simulink model "c_syst"  (R2015a)
settings: Solver=ode45  StartTime=0.0  StopTime=20  RelTol=1e-3
values from neighbouring files (symbols this model uses):
  A = A    [design.m]    (also in init.mat = [2.98564337206 1 0 0 0 -3.00327796547 0 1 0 0 0.709627661926)
  B = B    [design.m]    (also in init.mat = [1 0 0 0 0])
  C = [-0.0746143795197 0.142131862116 0 0 0]    [init.mat]
  D = zeros(1+length(A(:,1)),1)    [design.m]    (also in init.mat = 0)
  H = [C;eye(size(A))]    [design.m]
  Ke = -3.8587    [init.mat]
  Kp = 35.7244    [init.mat]
undefined symbols (not defined in the file or in its folder): K, M, National_Instruments, PCI
libraries: sldrtlib x2
settings Model: Creator=João  LastModifiedBy=João

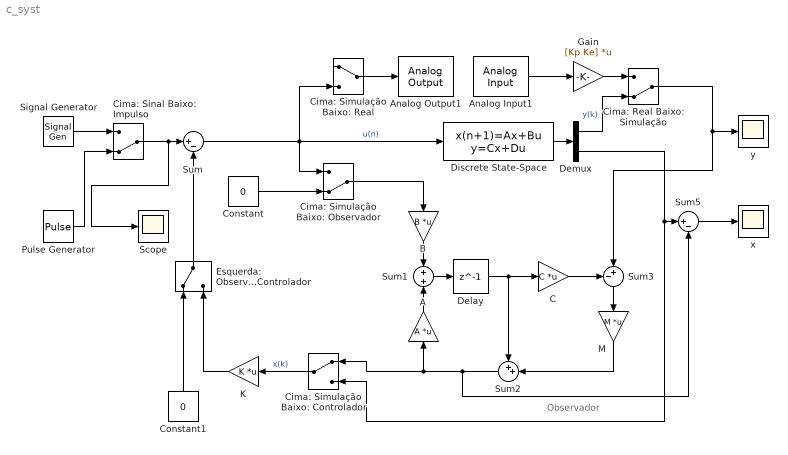
== system c_syst ==
  note: Observador
  A : Gain  Gain=A  Multiplication=Matrix(K*u) (u vector)
  Analog Input1 : sldrtlib/Analog Input  SampleTime=0.02  MaxMissedTicks=10  ShowMissedTicks=off  YieldWhenWaiting=off  DrvName=National_Instruments/PCI-6221  DrvAddress=4294967295  DrvOptions=[0 0 0 0 0]  Channels=[1 2]  RangeMode=1  VoltRange=1  DataType=1
      settings: AttributesFormatString=National Instruments\nPCI-6221 [auto]
  Analog Output1 : sldrtlib/Analog Output  SampleTime=0.02  MaxMissedTicks=10  ShowMissedTicks=off  YieldWhenWaiting=off  DrvName=National_Instruments/PCI-6221  DrvAddress=4294967295  DrvOptions=[0 0 0 0 0]  Channels=1  RangeMode=1  VoltRange=1  InitialValue=0  FinalValue=0
      settings: AttributesFormatString=National Instruments\nPCI-6221 [auto]
  B : Gain  Gain=B  Multiplication=Matrix(K*u) (u vector)
  C : Gain  Gain=C  Multiplication=Matrix(K*u) (u vector)
  Cima: Real Baixo: Simulação : ManualSwitch  CurrentSetting=0
  Cima: Simulação Baixo: Controlador : ManualSwitch
  Cima: Simulação Baixo: Observador : ManualSwitch  CurrentSetting=0
  Cima: Simulação Baixo: Real : ManualSwitch
  Cima: Sinal Baixo: Impulso : ManualSwitch  CurrentSetting=0
  Constant : Constant  Value=0
  Constant1 : Constant  Value=0
  Delay : Delay  DelayLength=1  InitialCondition=0  SampleTime=0.02
  Demux : Demux  Outputs=2
  Discrete State-Space : DiscreteStateSpace  A=A  B=B  C=H  D=D  SampleTime=0.02
  Esquerda: Observador Direita: Simulação e Controlador : ManualSwitch
  Gain : Gain  Gain=[Kp Ke]  Multiplication=Matrix(K*u) (u vector)
  K : Gain  Gain=K  Multiplication=Matrix(K*u) (u vector)
  M : Gain  Gain=M  Multiplication=Matrix(K*u) (u vector)
  Pulse Generator : DiscretePulseGenerator  PulseType=Time based  Period=20  PhaseDelay=2
  Scope : Scope
      settings: SampleInput=on
  Signal Generator : SignalGenerator  Units=rad/sec
  Sum : Sum  Inputs=|+-
  Sum1 : Sum  Inputs=+|+
  Sum2 : Sum  Inputs=++|
  Sum3 : Sum  Inputs=-+|
  Sum5 : Sum  Inputs=|+-
  x : Scope
      settings: SaveName=ScopeData2  SampleInput=on
  y : Scope
      settings: SampleInput=on
  wires:
  Sum/1 -> Cima: Simulação Baixo: Real/2, Cima: Simulação Baixo: Observador/1, Discrete State-Space/1  "u(n)"
  B/1 -> Sum1/1
  Sum1/1 -> Delay/1
  Sum2/1 -> Sum5/2, A/1, Cima: Simulação Baixo: Controlador/1
  A/1 -> Sum1/2
  Delay/1 -> C/1, Sum2/1
  C/1 -> Sum3/1
  Sum3/1 -> M/1
  M/1 -> Sum2/2
  Discrete State-Space/1 -> Demux/1
  Cima: Simulação Baixo: Controlador/1 -> K/1  "x(k)"
  Demux/2 -> Sum5/1, Cima: Simulação Baixo: Controlador/2
  Cima: Simulação Baixo: Observador/1 -> B/1
  Constant/1 -> Cima: Simulação Baixo: Observador/2
  Esquerda: Observador Direita: Simulação e Controlador/1 -> Sum/2
  K/1 -> Esquerda: Observador Direita: Simulação e Controlador/2
  Constant1/1 -> Esquerda: Observador Direita: Simulação e Controlador/1
  Cima: Sinal Baixo: Impulso/1 -> Scope/1, Sum/1
  Signal Generator/1 -> Cima: Sinal Baixo: Impulso/1
  Pulse Generator/1 -> Cima: Sinal Baixo: Impulso/2
  Sum5/1 -> x/1
  Gain/1 -> Cima: Real Baixo: Simulação/1
  Demux/1 -> Cima: Real Baixo: Simulação/2  "y(k)"
  Cima: Real Baixo: Simulação/1 -> Sum3/2, y/1
  Cima: Simulação Baixo: Real/1 -> Analog Output1/1
  Analog Input1/1 -> Gain/1
